simulink model "TCLab_Identification"  (Simulink 10.3)
settings: Solver=ode45  StartTime=0.0  StopTime=4000  FixedStep=0.1  RelTol=1e-3  EnableMultiTasking=on
PreLoadFcn:
  | variables
values from neighbouring files (symbols this model uses):
  Ts = 1    [stepDV.mat]    (also in stepMV.mat; step_MV.mat)
libraries: Process x1
settings Model: Creator=auto2  LastModifiedBy=thibaut  MultithreadedSim=on  ExtModeTrigMode=oneshot  ExtModeArmWhenConnect=off
settings DataIOCC: SaveOutput=off  SaveTime=off  SignalLoggingName=sigsOut
settings OptimizationCC: BooleanDataType=off  InitFltsAndDblsToZero=on
settings DebuggingCC: SaveWithParameterizedLinksMsg=none  SignalResolutionControl=TryResolveAllWithWarning  MultiTaskDSMMsg=warning  MultiTaskCondExecSysMsg=none  PregeneratedLibrarySubsystemCodeDiagnostic=none
settings HardwareCC: TargetUnknown=on
settings ConfigComp: CovSFcnEnable=off

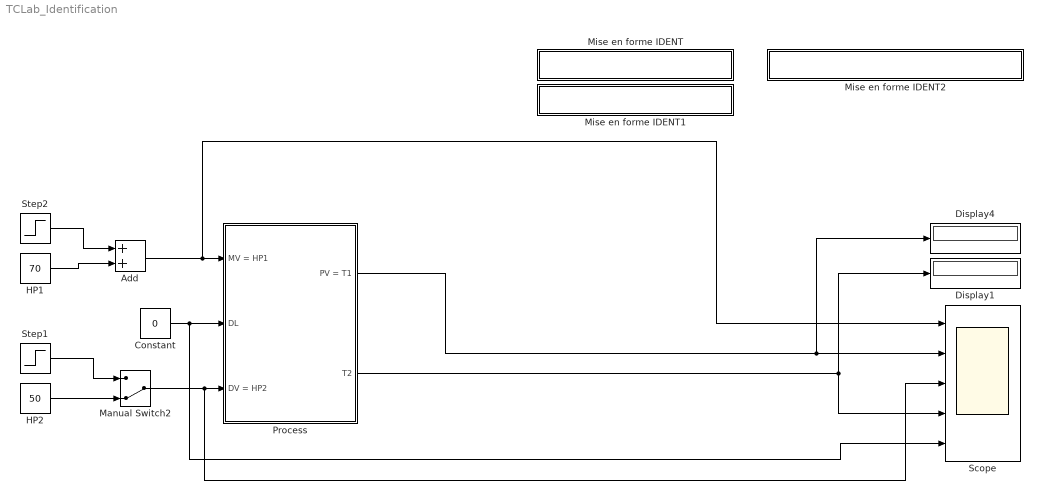
== system TCLab_Identification ==
  Add : Sum
  Constant : Constant  Value=0
  Display1 : Display
  Display4 : Display
  HP1 : Constant  Value=70  SampleTime=Ts
  HP2 : Constant  Value=50  SampleTime=Ts
  Manual Switch2 : ManualSwitch  CurrentSetting=0
  Mise en forme IDENT : Subsystem
      settings: OpenFcn=|
      | close all
      | 
      | t=ScopeData.time;
      | A=[ScopeData.signals.values];
      | u=A(:,1);
      | y=A(:,2);
      | 
      | figure(1)
      | subplot(211)
      | plot(t,u);
      | title('Original data: MV --> PV');
      | subplot(212)
      | plot(t,y);
      | grid
      | 
      | tstep=find(diff(u)~=0);
      | tstep=tstep(end);
      | 
      | y0 = y(tstep);
      | du = u(end)-u(tstep);
      | 
      | tm=t(tstep:end);
      | tm=tm-t(tstep);
      | um=u(tstep:end);
      | um=um-um(1);
      | ym=y(tstep:end);
      | ym=ym-ym(1);
      | 
      | ym = ym/(um(end));
      | um = um/(um(end));
      | 
      | figure(2)
      | subplot(211)
      | plot(tm,um);
      | title('Cleaned data for identification: MV --> PV');
      | subplot(212)
      | plot(tm,ym);
      | grid
      mask Display: disp('Prepare data MV = HP1 --> PV = T1')
  Mise en forme IDENT1 : Subsystem
      settings: OpenFcn=|
      | close all
      | 
      | t=ScopeData.time;
      | A=[ScopeData.signals.values];
      | u=A(:,3);
      | y=A(:,2);
      | 
      | figure(4)
      | subplot(211)
      | plot(t,u);
      | title('Original data: DV --> PV');
      | subplot(212)
      | plot(t,y);
      | grid
      | 
      | tstep=find(diff(u)~=0);
      | tstep=tstep(end);
      | 
      | y0 = y(tstep);
      | du = u(end)-u(tstep);
      | 
      | tm=t(tstep:end);
      | tm=tm-t(tstep);
      | um=u(tstep:end);
      | um=um-um(1);
      | ym=y(tstep:end);
      | ym=ym-ym(1);
      | 
      | ym = ym/(um(end));
      | um = um/(um(end));
      | 
      | figure(5)
      | subplot(211)
      | plot(tm,um);
      | title('Cleaned data for identification: DV --> PV');
      | subplot(212)
      | plot(tm,ym);
      | grid
      mask Display: disp('Prepare data DV = HP2 --> PV = T1')
  Mise en forme IDENT2 : Subsystem
      settings: OpenFcn=identification_fcn_VDG;
      mask Display: disp('IDENTIFICATION BASED ON PREPARED DATA')
  Process : Subsystem  BlockChoice=TCLab
      settings: AttributesFormatString=%<BlockChoice>  TemplateBlock=Process/Process  MemberBlocks=TCLab,TCLab_model
  Scope : Scope  NumInputPorts=5
  Step1 : Step  Time=300  Before=50  After=60  SampleTime=Ts
  Step2 : Step  Time=0  After=0  SampleTime=Ts
  wires:
  Manual Switch2/1 -> Process/3(DV = HP2), Scope/3
  Add/1 -> Scope/1, Process/1(MV = HP1)
  Process/1(PV = T1) -> Display4/1, Scope/2
  Process/2(T2) -> Scope/4, Display1/1
  Step1/1 -> Manual Switch2/1
  HP2/1 -> Manual Switch2/2
  Constant/1 -> Scope/5, Process/2(DL)
  Step2/1 -> Add/1
  HP1/1 -> Add/2

== system TCLab_Identification/Mise en forme IDENT ==

== system TCLab_Identification/Mise en forme IDENT1 ==

== system TCLab_Identification/Mise en forme IDENT2 ==

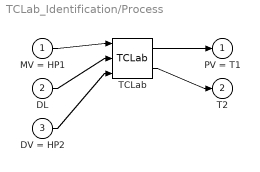
== system TCLab_Identification/Process ==
  MV = HP1 : Inport
  DL : Inport  Port=2
  DV = HP2 : Inport  Port=3
  TCLab : Process/TCLab  SystemSampleTime=-1  VariantActivationTime=update diagram  Latency=0  AutoFrameSizeCalculation=off
  PV = T1 : Outport  VectorParamsAs1DForOutWhenUnconnected=off
  T2 : Outport  Port=2  VectorParamsAs1DForOutWhenUnconnected=off
  wires:
  MV = HP1/1 -> TCLab/1
  DL/1 -> TCLab/2
  DV = HP2/1 -> TCLab/3
  TCLab/1 -> PV = T1/1
  TCLab/2 -> T2/1
